simulink model "controller"  (R2015a)
settings: Solver=ode3  StartTime=0.0  StopTime=5  FixedStep=0.1  RelTol=1e-3
libraries: fuzblock x2
settings Model: Creator=BML  LastModifiedBy=BML
settings SolverCC: AutoInsertRateTranBlk=on

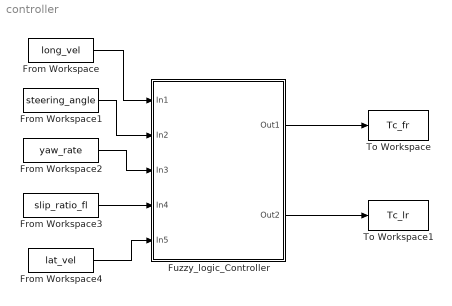
== system controller ==
  From Workspace : FromWorkspace  VariableName=long_vel  SampleTime=1
  From Workspace1 : FromWorkspace  VariableName=steering_angle  SampleTime=1
  From Workspace2 : FromWorkspace  VariableName=yaw_rate  SampleTime=1
  From Workspace3 : FromWorkspace  VariableName=slip_ratio_fl  SampleTime=1
  From Workspace4 : FromWorkspace  VariableName=lat_vel  SampleTime=1
  Fuzzy_logic_Controller : Subsystem
  To Workspace : ToWorkspace  VariableName=Tc_fr  SaveFormat=Timeseries  SampleTime=-1
  To Workspace1 : ToWorkspace  VariableName=Tc_lr  SaveFormat=Timeseries  SampleTime=-1
  wires:
  From Workspace/1 -> Fuzzy_logic_Controller/1(In1)
  From Workspace1/1 -> Fuzzy_logic_Controller/2(In2)
  From Workspace2/1 -> Fuzzy_logic_Controller/3(In3)
  From Workspace3/1 -> Fuzzy_logic_Controller/4(In4)
  From Workspace4/1 -> Fuzzy_logic_Controller/5(In5)
  Fuzzy_logic_Controller/1(Out1) -> To Workspace/1
  Fuzzy_logic_Controller/2(Out2) -> To Workspace1/1

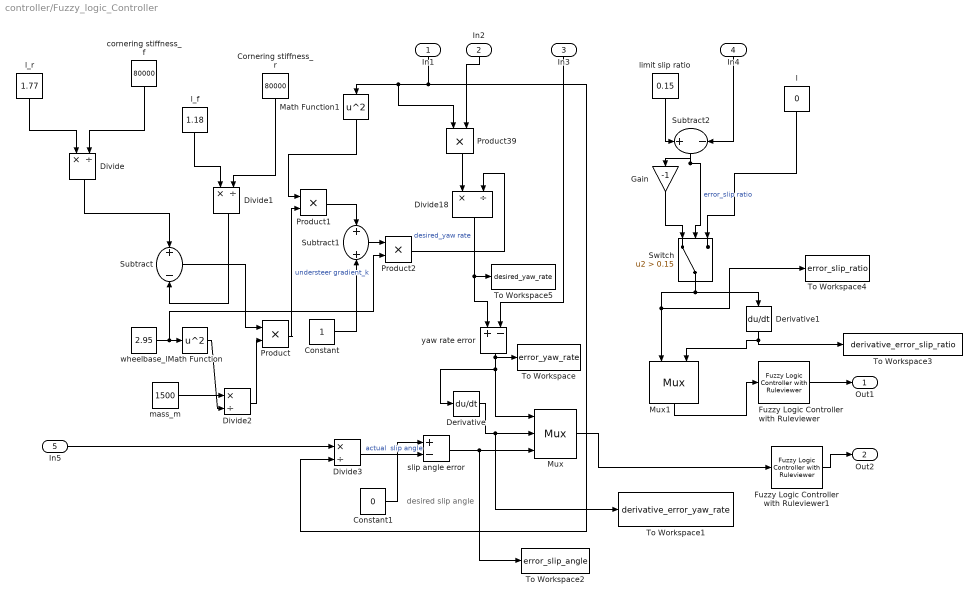
== system controller/Fuzzy_logic_Controller ==
  note: desired
      | slip angle
  In1 : Inport
  In2 : Inport  Port=2
  In3 : Inport  Port=3
  In4 : Inport  Port=4
  In5 : Inport  Port=5
  Constant : Constant
  Constant1 : Constant  Value=0
  "Cornering stiffness_r " : Constant  Value=80000
  Derivative : Derivative
  Derivative1 : Derivative
  Divide{,1..3,18} (5 alike) : Product  Inputs=*/
  Fuzzy Logic Controller with Ruleviewer : fuzblock/Fuzzy Logic  Controller  with Ruleviewer  fismatrix=fuzzy_slip_ratio  Ts=2
  Fuzzy Logic Controller with Ruleviewer1 : fuzblock/Fuzzy Logic  Controller  with Ruleviewer  fismatrix=fuzzy_yaw_rate  Ts=2
  Gain : Gain  Gain=-1
  Math Function : Math  Operator=square  SaturateOnIntegerOverflow=on
  Math Function1 : Math  Operator=square  SaturateOnIntegerOverflow=on
  Mux : Mux  Inputs=3
  Mux1 : Mux  Inputs=2
  Product{,1..2,39} (4 alike) : Product
  Subtract : Sum  Inputs=+-
  Subtract1 : Sum
  Subtract2 : Sum  Inputs=+-
  Switch : Switch  Criteria=u2 > Threshold  Threshold=0.15
  To Workspace : ToWorkspace  VariableName=error_yaw_rate  SaveFormat=Timeseries  SampleTime=1
  To Workspace1 : ToWorkspace  VariableName=derivative_error_yaw_rate  SaveFormat=Timeseries  SampleTime=1
  To Workspace2 : ToWorkspace  VariableName=error_slip_angle  SaveFormat=Timeseries  SampleTime=1
  To Workspace3 : ToWorkspace  VariableName=derivative_error_slip_ratio  SaveFormat=Timeseries  SampleTime=1
  To Workspace4 : ToWorkspace  VariableName=error_slip_ratio  SaveFormat=Timeseries  SampleTime=1
  To Workspace5 : ToWorkspace  VariableName=desired_yaw_rate  SaveFormat=Timeseries  SampleTime=1
  "cornering stiffness_f " : Constant  Value=80000
  l : Constant  Value=0
  "l_f " : Constant  Value=1.18
  "l_r " : Constant  Value=1.77
  limit slip ratio : Constant  Value=0.15
  mass_m : Constant  Value=1500
  "slip angle error  " : Sum  Inputs=+-
  wheelbase_l : Constant  Value=2.95
  "yaw rate error   " : Sum  Inputs=+-
  Out1 : Outport
  Out2 : Outport  Port=2
  wires:
  Fuzzy Logic Controller with Ruleviewer/1 -> Out1/1
  Divide/1 -> Subtract/1
  Subtract/1 -> Product/1
  Product/1 -> Product1/2  "understeer gradient_k"
  Constant/1 -> Subtract1/2
  Product39/1 -> Divide18/1
  Product2/1 -> Divide18/2
  In2/1 -> Product39/2
  Math Function1/1 -> Product1/1
  Subtract1/1 -> Product2/1
  In5/1 -> Divide3/1
  "l_r "/1 -> Divide/1
  Divide1/1 -> Subtract/2
  "Cornering stiffness_r "/1 -> Divide1/2
  wheelbase_l/1 -> Product2/2, Math Function/1
  mass_m/1 -> Divide2/1
  Math Function/1 -> Divide2/2
  Divide2/1 -> Product/2
  In1/1 -> Divide3/2, Math Function1/1, Product39/1
  "l_f "/1 -> Divide1/1
  "cornering stiffness_f "/1 -> Divide/2
  Product1/1 -> Subtract1/1
  Constant1/1 -> "slip angle error  "/1
  Switch/1 -> Mux1/1, To Workspace4/1, Derivative1/1
  In3/1 -> "yaw rate error   "/2
  Divide18/1 -> To Workspace5/1, "yaw rate error   "/1  "desired_yaw rate"
  Subtract2/1 -> Switch/2, Gain/1  "error_slip ratio"
  Gain/1 -> Switch/1
  limit slip ratio/1 -> Subtract2/1
  Derivative/1 -> To Workspace1/1, Mux/2
  Mux/1 -> Fuzzy Logic Controller with Ruleviewer1/1
  In4/1 -> Subtract2/2
  l/1 -> Switch/3
  Divide3/1 -> "slip angle error  "/2  "actual  slip angle"
  "slip angle error  "/1 -> To Workspace2/1, Mux/3
  Derivative1/1 -> Mux1/2, To Workspace3/1
  Mux1/1 -> Fuzzy Logic Controller with Ruleviewer/1
  Fuzzy Logic Controller with Ruleviewer1/1 -> Out2/1
  "yaw rate error   "/1 -> To Workspace/1, Mux/1, Derivative/1
